simulink model "BlockDiagram"  (R2020a)
settings: Solver=FixedStepAuto  StartTime=0.0  StopTime=7.5  FixedStep=0.005  RelTol=1e-3
values from neighbouring files (symbols this model uses):
  Kc = 01.0097390    (= 1.009739)    [InputDesign.m]
  Kr = 495.7373    [InputDesign.m]
  T1 = 0.005077    [InputDesign.m]
  Tr = 0.01063    [InputDesign.m]
undefined symbols (not defined in the file or in its folder): Efd0, K_S1, K_S2, K_S3, T_1, T_10, T_11, T_2, T_3, T_4, T_6, T_7, T_8, T_9, T_w1, T_w2, T_w3, T_w4, V_S1MAX, V_S1MIN, V_S2MAX, V_S2MIN, V_STMAX, V_STMIN, Vinit, VR0, Vrmax, Vrmin, XadIfd
libraries: eeGeneralControl x4, simulink x1, fmu_me_lib x1
settings Model: Creator=meagh

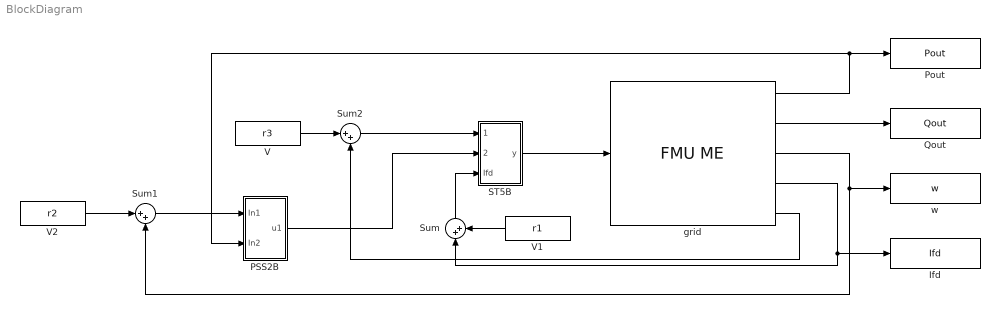
== system BlockDiagram ==
  Ifd : ToWorkspace  VariableName=Ifd  SaveFormat=Timeseries  SampleTime=-1
  PSS2B : Subsystem
  Pout : ToWorkspace  VariableName=Pout  SaveFormat=Timeseries  SampleTime=-1
  Qout : ToWorkspace  VariableName=Qout  SaveFormat=Timeseries  SampleTime=-1
  ST5B : Subsystem
  Sum : Sum  Inputs=|++
  Sum1 : Sum  Inputs=|++
  Sum2 : Sum  Inputs=|++
  V : FromWorkspace  VariableName=r3
  V1 : FromWorkspace  VariableName=r1
  V2 : FromWorkspace  VariableName=r2
  grid : fmu_me_lib/FMU ME  Description=Simulates an FMU for Model Exchange 1.0 or Model Exchange 2.0.  dummy=0
  w : ToWorkspace  VariableName=w  SaveFormat=Timeseries  SampleTime=-1
  wires:
  PSS2B/1(u1) -> ST5B/2(VOTHSG)
  ST5B/1(y) -> grid/1
  grid/1 -> Pout/1, PSS2B/2(In2)
  grid/3 -> Sum1/2, w/1
  grid/2 -> Qout/1
  Sum/1 -> ST5B/3(Ifd)
  grid/4 -> Ifd/1, Sum/1
  V1/1 -> Sum/2
  Sum1/1 -> PSS2B/1(In1)
  V2/1 -> Sum1/1
  V/1 -> Sum2/1
  Sum2/1 -> ST5B/1(Ecomp)
  grid/5 -> Sum2/2

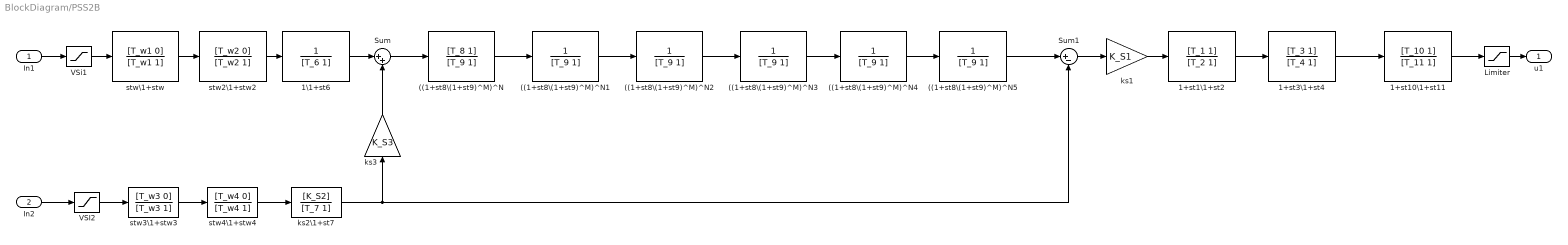
== system BlockDiagram/PSS2B ==
  In1 : Inport
  In2 : Inport  Port=2
  ((1+st8\(1+st9)^M)^N : TransferFcn  Numerator=[T_8 1]  Denominator=[T_9 1]
  ((1+st8\(1+st9)^M)^N{1..5} (5 alike) : TransferFcn  Denominator=[T_9 1]
  1+st10\1+st11 : TransferFcn  Numerator=[T_10 1]  Denominator=[T_11 1]
  1+st1\1+st2 : TransferFcn  Numerator=[T_1 1]  Denominator=[T_2 1]
  1+st3\1+st4 : TransferFcn  Numerator=[T_3 1]  Denominator=[T_4 1]
  1\1+st6 : TransferFcn  Denominator=[T_6 1]
  "Limiter " : Saturate  UpperLimit=V_STMAX  LowerLimit=V_STMIN
  Sum : Sum  Inputs=|++
  Sum1 : Sum  Inputs=|+-
  VSI2 : Saturate  UpperLimit=V_S2MAX  LowerLimit=V_S2MIN
  VSi1 : Saturate  UpperLimit=V_S1MAX  LowerLimit=V_S1MIN
  ks1 : Gain  Gain=K_S1  SaturateOnIntegerOverflow=on  OutDataTypeStr=Inherit: Same as input  ParamDataTypeStr=Inherit: Same as input
  ks2\1+st7 : TransferFcn  Numerator=[K_S2]  Denominator=[T_7 1]
  ks3 : Gain  Gain=K_S3  SaturateOnIntegerOverflow=on  OutDataTypeStr=Inherit: Same as input  ParamDataTypeStr=Inherit: Same as input
  stw2\1+stw2 : TransferFcn  Numerator=[T_w2 0]  Denominator=[T_w2 1]
  stw3\1+stw3 : TransferFcn  Numerator=[T_w3 0]  Denominator=[T_w3 1]
  stw4\1+stw4 : TransferFcn  Numerator=[T_w4 0]  Denominator=[T_w4 1]
  stw\1+stw : TransferFcn  Numerator=[T_w1 0]  Denominator=[T_w1 1]
  u1 : Outport
  wires:
  1+st3\1+st4/1 -> 1+st10\1+st11/1
  ((1+st8\(1+st9)^M)^N4/1 -> ((1+st8\(1+st9)^M)^N5/1
  ((1+st8\(1+st9)^M)^N2/1 -> ((1+st8\(1+st9)^M)^N3/1
  ((1+st8\(1+st9)^M)^N/1 -> ((1+st8\(1+st9)^M)^N1/1
  1\1+st6/1 -> Sum/1
  stw2\1+stw2/1 -> 1\1+st6/1
  Sum1/1 -> ks1/1
  ((1+st8\(1+st9)^M)^N1/1 -> ((1+st8\(1+st9)^M)^N2/1
  ks3/1 -> Sum/2
  In1/1 -> VSi1/1
  VSI2/1 -> stw3\1+stw3/1
  ((1+st8\(1+st9)^M)^N5/1 -> Sum1/1
  Sum/1 -> ((1+st8\(1+st9)^M)^N/1
  1+st1\1+st2/1 -> 1+st3\1+st4/1
  VSi1/1 -> stw\1+stw/1
  1+st10\1+st11/1 -> "Limiter "/1
  ks1/1 -> 1+st1\1+st2/1
  ((1+st8\(1+st9)^M)^N3/1 -> ((1+st8\(1+st9)^M)^N4/1
  ks2\1+st7/1 -> Sum1/2, ks3/1
  stw\1+stw/1 -> stw2\1+stw2/1
  stw4\1+stw4/1 -> ks2\1+st7/1
  stw3\1+stw3/1 -> stw4\1+stw4/1
  In2/1 -> VSI2/1
  "Limiter "/1 -> u1/1

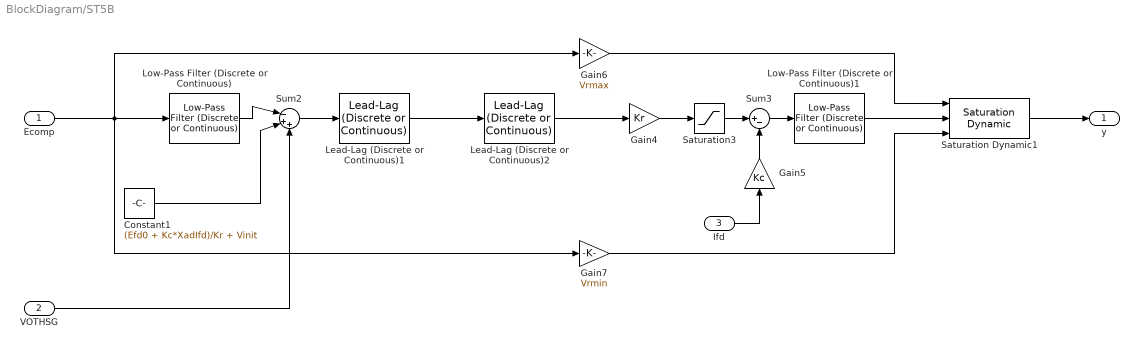
== system BlockDiagram/ST5B ==
  Ecomp : Inport
  VOTHSG : Inport  Port=2
  Ifd : Inport  Port=3
  Constant1 : Constant  Value=(Efd0 + Kc*XadIfd)/Kr + Vinit
  Gain4 : Gain  Gain=Kr
  Gain5 : Gain  Gain=Kc
  Gain6 : Gain  Gain=Vrmax
  Gain7 : Gain  Gain=Vrmin
  Lead-Lag (Discrete or Continuous)1 : eeGeneralControl/Lead-Lag (Discrete or Continuous)  T1=Tb1  T2=Tc1  B=Vrmax/Kr  A=Vrmin/Kr  init_option=Inherited from block input  x0=VR0/Kr  Ts=0
      settings: SourceProductBaseCode=PS
  Lead-Lag (Discrete or Continuous)2 : eeGeneralControl/Lead-Lag (Discrete or Continuous)  T1=Tb2  T2=Tc2  B=Vrmax/Kr  A=Vrmin/Kr  init_option=Inherited from block input  x0=VR0/Kr  Ts=0
      settings: SourceProductBaseCode=PS
  Low-Pass Filter (Discrete or Continuous) : eeGeneralControl/Low-Pass Filter (Discrete or Continuous)  K=1  T=Tr  B=inf  A=-inf  init_option=Inherited from block input  x0=0  Ts=0
  Low-Pass Filter (Discrete or Continuous)1 : eeGeneralControl/Low-Pass Filter (Discrete or Continuous)  K=1  T=T1  B=inf  A=-inf  init_option=Inherited from block input  x0=0  Ts=0
  Saturation Dynamic1 : simulink/Discontinuities/Saturation Dynamic  OutMin=[]  OutMax=[]  OutDataTypeStr=Inherit: Same as second input  OutDataType=fixdt(1, 16)  OutScaling=2^-10  DoSatur=off
  Saturation3 : Saturate  UpperLimit=Vrmax  LowerLimit=Vrmin  LinearizeAsGain=off
  Sum2 : Sum  Inputs=|-++
  Sum3 : Sum  Inputs=|+-
  y : Outport
  wires:
  Gain6/1 -> Saturation Dynamic1/1
  Sum3/1 -> Low-Pass Filter (Discrete or Continuous)1/1
  Lead-Lag (Discrete or Continuous)2/1 -> Gain4/1
  Ecomp/1 -> Low-Pass Filter (Discrete or Continuous)/1, Gain7/1, Gain6/1
  Saturation3/1 -> Sum3/1
  Gain5/1 -> Sum3/2
  Constant1/1 -> Sum2/2
  Gain7/1 -> Saturation Dynamic1/3
  Ifd/1 -> Gain5/1
  Low-Pass Filter (Discrete or Continuous)1/1 -> Saturation Dynamic1/2
  Gain4/1 -> Saturation3/1
  Low-Pass Filter (Discrete or Continuous)/1 -> Sum2/1
  Sum2/1 -> Lead-Lag (Discrete or Continuous)1/1
  Lead-Lag (Discrete or Continuous)1/1 -> Lead-Lag (Discrete or Continuous)2/1
  Saturation Dynamic1/1 -> y/1
  VOTHSG/1 -> Sum2/3
